simulink model "dsPIC33CK256MP508_MCLV2_SMO_Motor"  (R2022a)
settings: Solver=FixedStepDiscrete  StartTime=0.0  StopTime=10  FixedStep=.00005  RelTol=1e-3  EnableMultiTasking=on
InitFcn:
  | dsPIC33CK256MP508_MCLV2_SMO_data;
values from neighbouring files (symbols this model uses):
  PI_params = mcb.internal.SetControllerParameters(pmsm,inverter,PU_System,T_pwm,2*Ts,Ts_speed)    [dsPIC33CK256MP508_MCLV2_Generator_data.m]    (also in dsPIC33CK256MP508_MCLV2_SMO_data.m = mcb.internal.SetControllerParameters(pmsm,inverter,PU_System; mcb_pmsm_foc_qep_dsPIC33_data.m)
  PU_System = mcb_SetPUSystem(pmsm,inverter)    [dsPIC33CK256MP508_MCLV2_Generator_data.m]    (also in dsPIC33CK256MP508_MCLV2_SMO_data.m; mcb_pmsm_foc_qep_dsPIC33_data.m)
  PWM_frequency = 20e3    (= 20000)    [dsPIC33CK256MP508_MCLV2_Generator_data.m]    (also in dsPIC33CK256MP508_MCLV2_SMO_data.m; mcb_pmsm_foc_qep_dsPIC33_data.m)
  Speed_openLoop = 500    [dsPIC33CK256MP508_MCLV2_SMO_data.m]
  Ts = T_pwm    (= 5e-05)    [dsPIC33CK256MP508_MCLV2_Generator_data.m]    (also in dsPIC33CK256MP508_MCLV2_SMO_data.m; mcb_pmsm_foc_qep_dsPIC33_data.m)
  Ts_speed = 10*Ts    (= 0.0005)    [dsPIC33CK256MP508_MCLV2_Generator_data.m]    (also in dsPIC33CK256MP508_MCLV2_SMO_data.m = 0.0015; mcb_pmsm_foc_qep_dsPIC33_data.m)
undefined symbols (not defined in the file or in its folder): AN1, B0, B2, C9, D6, DiscIntNeverNeededParam, inverter, MaxPer, mcb_isCodeGenVar, mcb_isSimVar, P32, P57, P70, Pin, pmsm, PWM1max, Resol, s, us
libraries: MCHP_Blockset x13, simulink x10, mcbcontrolslib x9, slpidlib x3
(part 3 of 3)

== system dsPIC33CK256MP508_MCLV2_SMO_Motor/Current Control/Input Scaling/Sliding Mode Observer/smo/atan2 ==
  note: Consistent with Microchip notation:
      |
      | x_α = cos(θ) * x_d - sin(θ) * x_q
      | x_β = sin(θ) * x_d + cos(θ) * x_q
      |
      | θ = atan2(sin(θ)/cos(θ)) = atan2(-x_α/x_β)
      |
      | provided x_d = 0, which is true in case of E_d
  α : Inport
  β : Inport  Port=2
  Bias2 : Bias  Bias=(pi/4)-(pi/25)  SaturateOnIntegerOverflow=off
  Data Type Conversion3 : DataTypeConversion  OutDataTypeStr=fixdt(1,16,12)  SaturateOnIntegerOverflow=off  RndMeth=Floor
  Data Type Conversion4 : DataTypeConversion  OutDataTypeStr=uint16  ConvertRealWorld=Stored Integer (SI)  SaturateOnIntegerOverflow=off  RndMeth=Floor
  Gain2 : Gain  Gain=1/2^12  OutDataTypeStr=fixdt(1,16,12)
  Gain3 : Gain  Gain=-1  OutDataTypeStr=Inherit: Same as input
  Subsystem1 : Subsystem
  Trigonometric Function : Trigonometry  Operator=atan2  ApproximationMethod=CORDIC
  Wrap_to_pi1 : Subsystem  VariantControl=VSS_STD
  θ : Outport  VectorParamsAs1DForOutWhenUnconnected=off
  wires:
  Trigonometric Function/1 -> Data Type Conversion3/1
  Gain3/1 -> Trigonometric Function/1
  α/1 -> Gain3/1
  β/1 -> Trigonometric Function/2
  Data Type Conversion3/1 -> Subsystem1/1(theta(-pi,pi))
  Subsystem1/1(theta(0,2pi)) -> Bias2/1
  Bias2/1 -> Data Type Conversion4/1
  Data Type Conversion4/1 -> Wrap_to_pi1/1(θ)
  Wrap_to_pi1/1(θ (0,2π)) -> Gain2/1  "z"
  Gain2/1 -> θ/1

== system dsPIC33CK256MP508_MCLV2_SMO_Motor/Current Control/Input Scaling/Sliding Mode Observer/smo/Subsystem/Wrap_to_pi2 ==
  note: What's left after
      | division by 2pi
  note: This block limits the output angle between +/- π.
  note: Add pi
  note: What's left after
      | division by 2pi
      | again
  note: Subtract pi
  θ : Inport
  Bias : Bias  Bias=pi*16777216  SaturateOnIntegerOverflow=off
  Bias1 : Bias  Bias=-pi*16777216  SaturateOnIntegerOverflow=off
  Math Function : Math  Operator=mod  SignedPower=on
  Math Function1 : Math  Operator=mod  SignedPower=on
  load torque1 : Constant  Value=2*pi*16777216  OutDataTypeStr=int32  SampleTime=Ts
  θ (-π,π) : Outport  VectorParamsAs1DForOutWhenUnconnected=off
  wires:
  Math Function1/1 -> Bias/1
  θ/1 -> Math Function1/1
  Math Function/1 -> Bias1/1
  load torque1/1 -> Math Function1/2, Math Function/2
  Bias/1 -> Math Function/1
  Bias1/1 -> θ (-π,π)/1

== system dsPIC33CK256MP508_MCLV2_SMO_Motor/Current Control/Input Scaling/Sliding Mode Observer/smo/atan2/Subsystem1 ==
  theta(-pi,pi) : Inport
  2pi : Constant  Value=2*pi  OutDataTypeStr=fixdt(1,16,12)  SampleTime=Ts  mask(TL_Constant){data={'date',734873.5078369329}}
      settings: CopyFcn=if exist('tl_reset_reviewflag','file')==2,tl_reset_reviewflag(gcbh);end  DeleteFcn=if exist('delete_tlblock','file')==2,delete_tlblock(gcbh);end  NameChangeFcn=if exist('rename_tlblock','file')==2,rename_tlblock(gcbh);end  OpenFcn=if exist('tl_open_blockdlg','file')==2,tl_open_blockdlg(gcbh);else,open_system(gcbh,'parameter');end
      mask Help: eval(['if exist(''tl_online_help'',''file'') == 2, tl_online_help(''Topic'',''TL_Constant''),else, web([''jar:file:///'',matlabroot,''/help/toolbox/simulink/help.jar!/slref/' lower(get_param(gcbh,'Blocktype')) '.html''], ''-helpbrowser''),end'])
      mask Display: plot([-0.05, 1.05, NaN, -0.05, 1.05],[.01, .01, NaN, .99, .99])
  Sum : Sum
  Switch2 : Switch  Criteria=u2 > Threshold  SaturateOnIntegerOverflow=off  InputSameDT=off
  theta(0,2pi) : Outport  VectorParamsAs1DForOutWhenUnconnected=off
  wires:
  2pi/1 -> Sum/2
  theta(-pi,pi)/1 -> Sum/1, Switch2/2, Switch2/1
  Sum/1 -> Switch2/3  "err"
  Switch2/1 -> theta(0,2pi)/1

== system dsPIC33CK256MP508_MCLV2_SMO_Motor/Current Control/Input Scaling/Sliding Mode Observer/smo/atan2/Wrap_to_pi1 ==
  note: This block limits the output angle between 0 to 2π.
  θ : Inport
  Math Function : Math  Operator=rem  SignedPower=on
  load torque2 : Constant  Value=2*pi*2^12  OutDataTypeStr=uint16  SampleTime=Ts
  θ (0,2π) : Outport  VectorParamsAs1DForOutWhenUnconnected=off
  wires:
  Math Function/1 -> θ (0,2π)/1
  θ/1 -> Math Function/1
  load torque2/1 -> Math Function/2

== stateflow chart dsPIC33CK256MP508_MCLV2_SMO_Motor/Current Control/Input Scaling/OpentoClosed/Chart ==
  state Init
    during: Mode = 0;
    SpeedCtrl == 0;
  state Align
    during: Mode = 0;
    SpeedCtrl == 0;
  state ClosedLoopFilter
    during: Mode = 2;
    SpeedCtrl == 1;
  state ClosedLoop
    during: Mode = 2;
    SpeedCtrl == 0;
  state OpenLoop
    during: Mode = 1;
    SpeedCtrl == 0;
  (default) -> Init
  ClosedLoopFilter -> Init : [En == 0]
  ClosedLoop -> Init [order 1] : [En == 0]
  Init -> Align : [En == 1]
  Align -> Init [order 1] : [En == 0]
  OpenLoop -> Init [order 2] : [En == 0]
  Align -> OpenLoop [order 2] : after(0.5,sec)
  ClosedLoop -> ClosedLoopFilter [order 2] : after(0.1,sec)
  OpenLoop -> ClosedLoop [order 1] : after(2,sec)[SpeedFb > Limit]
  data: Limit input fixdt(1,16,14); SpeedFb input fixdt(1,16,14); Mode output uint16; En input boolean; SpeedCtrl output boolean
